simulink model "AsteroidImpact"  (R2020a)
settings: Solver=ode4  StartTime=0.0  StopTime=200  FixedStep=0.2  RelTol=1e-3
values from neighbouring files (symbols this model uses):
  K1 = 1.0e+03 *[-1.1353   -0.0611    0.0001   -0.0000;-0.0000   -0.0000    0.0000    1.0000]    [define_constants.m]    (also in setup_controller.m)
  K2 = 1.0e+03 *[-2.9174   -0.3964    0.0027    0.0000;0.0000    0.0000   -0.0000    0.0800]    [define_constants.m]    (also in setup_controller.m)
  MASS = 1000    [define_constants.m]
settings Model: Creator=KNMALE002  LastModifiedBy=Flaz
settings DataIOCC: SaveOutput=off  SignalLogging=off  DSMLogging=off  ReturnWorkspaceOutputs=off  TimeSaveName=simulation_time
settings DebuggingCC: ArithmeticOperatorsInVariantConditions=warning
settings SFSimCC: CustomCodeUndefinedFunction=UseInterfaceOnly

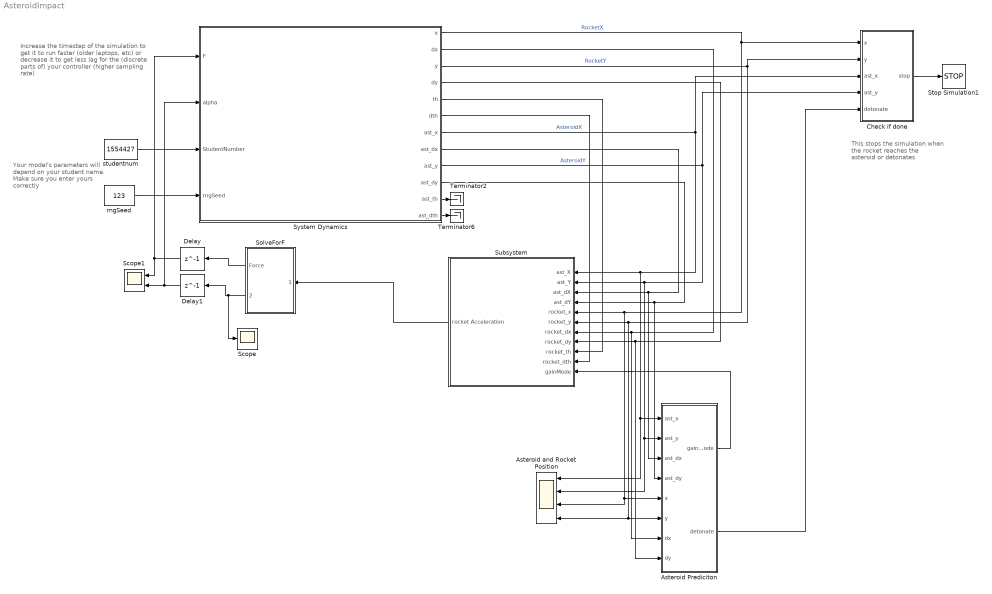
== system AsteroidImpact ==
  note: Increase the timestep of the simulation to get it to run faster (older laptops, etc) or decrease it to get less lag for the (discrete parts of) your controller (higher sampling rate)
  note: Your model's parameters will depend on your student name. Make sure you enter yours correctly
  note: This stops the simulation when the rocket reaches the asteroid or detonates
  Asteroid Prediciton : MATLAB Function  TreatAsAtomicUnit=on
  Asteroid and Rocket Position : Scope  NumInputPorts=4
  Check if done : MATLAB Function  TreatAsAtomicUnit=on
  Delay : Delay  DelayLength=1  InitialCondition=10000000000
  Delay1 : Delay  DelayLength=1
  Scope : Scope
  Scope1 : Scope  NumInputPorts=2
  SolveForF : MATLAB Function  TreatAsAtomicUnit=on
  Stop Simulation1 : Stop
  Subsystem : Subsystem
  System Dynamics : Subsystem  TreatAsAtomicUnit=on  mask{Value=2}
      mask prompts: Value "Enter mode (1, 2 or 3)"
      mask TypeOptions Value: ScenarioVar/Value
      mask Display: image('lander.jpg');
  Terminator2 : Terminator
  Terminator6 : Terminator
  rngSeed : Constant  Value=123
  studentnum : Constant  Value=1554427
  wires:
  studentnum/1 -> System Dynamics/3(StudentNumber)
  rngSeed/1 -> System Dynamics/4(rngSeed)
  System Dynamics/12(ast_dth) -> Terminator6/1
  System Dynamics/11(ast_th) -> Terminator2/1
  Check if done/1(stop) -> Stop Simulation1/1
  Delay1/1 -> Scope1/2, System Dynamics/2(alpha)
  Delay/1 -> Scope1/1, System Dynamics/1(F)
  System Dynamics/10(ast_dy) -> Asteroid Prediciton/4(ast_dy), Subsystem/4(ast_dY)
  SolveForF/1(Force) -> Delay/1
  SolveForF/2(angleAlpha) -> Scope/1, Delay1/1
  System Dynamics/1(x) -> Asteroid and Rocket Position/3, Asteroid Prediciton/5(x), Subsystem/5(rocket_x), Check if done/1(x)  "RocketX"
  System Dynamics/7(ast_x) -> Check if done/3(ast_x), Subsystem/1(ast_X), Asteroid Prediciton/1(ast_x), Asteroid and Rocket Position/1  "AsteroidX"
  System Dynamics/9(ast_y) -> Check if done/4(ast_y), Asteroid and Rocket Position/2, Asteroid Prediciton/2(ast_y), Subsystem/2(ast_Y)  "AsteroidY"
  System Dynamics/8(ast_dx) -> Asteroid Prediciton/3(ast_dx), Subsystem/3(ast_dX)
  System Dynamics/4(dy) -> Subsystem/8(rocket_dy), Asteroid Prediciton/8(dy)
  System Dynamics/2(dx) -> Asteroid Prediciton/7(dx), Subsystem/7(rocket_dx)
  System Dynamics/3(y) -> Check if done/2(y), Asteroid and Rocket Position/4, Asteroid Prediciton/6(y), Subsystem/6(rocket_y)  "RocketY"
  System Dynamics/5(th) -> Subsystem/9(rocket_th)
  System Dynamics/6(dth) -> Subsystem/10(rocket_dth)
  Subsystem/1(rocket Acceleration) -> SolveForF/1(rocketAcceleration)
  Asteroid Prediciton/1(gainMode) -> Subsystem/11(gainMode)
  Asteroid Prediciton/2(detonate) -> Check if done/5(detonate)

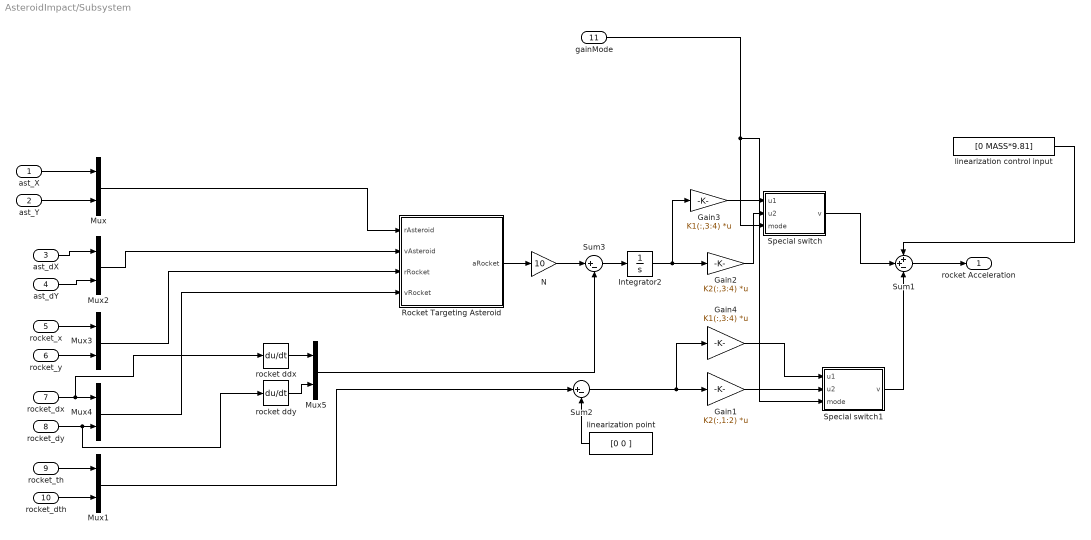
== system AsteroidImpact/Subsystem ==
  ast_X : Inport
  ast_Y : Inport  Port=2
  ast_dX : Inport  Port=3
  ast_dY : Inport  Port=4
  rocket_x : Inport  Port=5
  rocket_y : Inport  Port=6
  rocket_dx : Inport  Port=7
  rocket_dy : Inport  Port=8
  rocket_th : Inport  Port=9
  rocket_dth : Inport  Port=10
  gainMode : Inport  Port=11
  Gain1 : Gain  Gain=K2(:,1:2)  Multiplication=Matrix(K*u)
  Gain2 : Gain  Gain=K2(:,3:4)  Multiplication=Matrix(K*u)
  Gain3 : Gain  Gain=K1(:,3:4)  Multiplication=Matrix(K*u)
  Gain4 : Gain  Gain=K1(:,3:4)  Multiplication=Matrix(K*u)
  Integrator2 : Integrator
  Mux{,1..5} (6 alike) : Mux  Inputs=2
  N : Gain  Gain=10
  Rocket Targeting Asteroid : MATLAB Function  TreatAsAtomicUnit=on
  Special switch : MATLAB Function  TreatAsAtomicUnit=on
  Special switch1 : MATLAB Function  TreatAsAtomicUnit=on
  Sum1 : Sum  Inputs=++-
  Sum2 : Sum  Inputs=|+-
  Sum3 : Sum  Inputs=|+-
  linearization control input : Constant  Value=[0 MASS*9.81]
  linearization point : Constant  Value=[0 0 ]
  rocket ddx : Derivative
  rocket ddy : Derivative
  rocket Acceleration : Outport
  wires:
  Mux5/1 -> Sum3/2
  rocket_x/1 -> Mux3/1
  Sum3/1 -> Integrator2/1
  Mux2/1 -> Rocket Targeting Asteroid/2(vAsteroid)
  ast_X/1 -> Mux/1
  ast_Y/1 -> Mux/2
  ast_dX/1 -> Mux2/1
  ast_dY/1 -> Mux2/2
  rocket_dy/1 -> rocket ddy/1, Mux4/2
  rocket ddy/1 -> Mux5/2
  rocket_dx/1 -> rocket ddx/1, Mux4/1
  Rocket Targeting Asteroid/1(aRocket) -> N/1
  N/1 -> Sum3/1
  rocket ddx/1 -> Mux5/1
  rocket_y/1 -> Mux3/2
  Sum2/1 -> Gain4/1, Gain1/1
  Integrator2/1 -> Gain3/1, Gain2/1
  linearization point/1 -> Sum2/2
  Sum1/1 -> rocket Acceleration/1
  Mux3/1 -> Rocket Targeting Asteroid/3(rRocket)
  rocket_dth/1 -> Mux1/2
  rocket_th/1 -> Mux1/1
  linearization control input/1 -> Sum1/1
  Mux4/1 -> Rocket Targeting Asteroid/4(vRocket)
  Mux/1 -> Rocket Targeting Asteroid/1(rAsteroid)
  Mux1/1 -> Sum2/1
  Special switch/1(v) -> Sum1/2
  Gain2/1 -> Special switch/2(u2)
  Gain3/1 -> Special switch/1(u1)
  gainMode/1 -> Special switch1/3(mode), Special switch/3(mode)
  Special switch1/1(v) -> Sum1/3
  Gain1/1 -> Special switch1/2(u2)
  Gain4/1 -> Special switch1/1(u1)

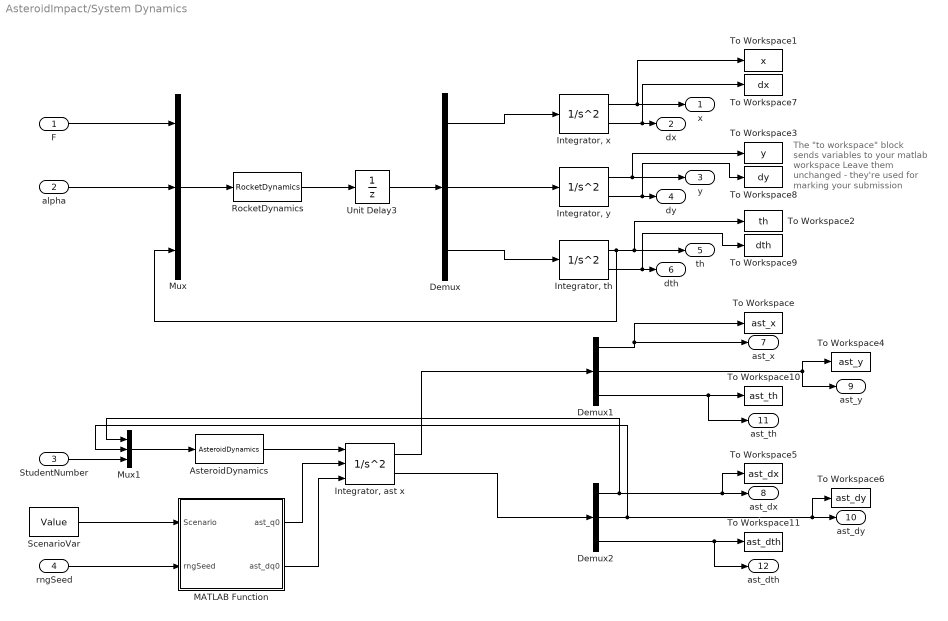
== system AsteroidImpact/System Dynamics ==
  note: The "to workspace" block sends variables to your matlab workspace
      |
      | Leave them unchanged - they're used for marking your submission
  F : Inport
  alpha : Inport  Port=2
  StudentNumber : Inport  Port=3
  rngSeed : Inport  Port=4
  AsteroidDynamics : MATLABFcn  MATLABFcn=AsteroidDynamics  OutputDimensions=3
  Demux : Demux  Outputs=3
  Demux1 : Demux  Outputs=3
  Demux2 : Demux  Outputs=3
  "Integrator, th" : SecondOrderIntegrator  ICX=0  ICDXDT=0
  "Integrator, x" : SecondOrderIntegrator  ICX=0
  "Integrator, y" : SecondOrderIntegrator  ICX=0
  "Integrator, ast x" : SecondOrderIntegrator  ICSourceX=external  ICX=x0  ICSourceDXDT=external
  MATLAB Function : MATLAB Function  TreatAsAtomicUnit=on
  Mux : Mux  Inputs=3
  Mux1 : Mux  Inputs=3
  RocketDynamics : MATLABFcn  MATLABFcn=RocketDynamics  Output1D=off
  ScenarioVar : Constant  Value=Value
  To Workspace : ToWorkspace  VariableName=ast_x  SampleTime=-1
  To Workspace1 : ToWorkspace  VariableName=x  SampleTime=-1
  To Workspace10 : ToWorkspace  VariableName=ast_th  SampleTime=-1
  To Workspace11 : ToWorkspace  VariableName=ast_dth  SampleTime=-1
  To Workspace2 : ToWorkspace  VariableName=th  SampleTime=-1
  To Workspace3 : ToWorkspace  VariableName=y  SampleTime=-1
  To Workspace4 : ToWorkspace  VariableName=ast_y  SampleTime=-1
  To Workspace5 : ToWorkspace  VariableName=ast_dx  SampleTime=-1
  To Workspace6 : ToWorkspace  VariableName=ast_dy  SampleTime=-1
  To Workspace7 : ToWorkspace  VariableName=dx  SampleTime=-1
  To Workspace8 : ToWorkspace  VariableName=dy  SampleTime=-1
  To Workspace9 : ToWorkspace  VariableName=dth  SampleTime=-1
  Unit Delay3 : UnitDelay  SampleTime=-1  HasFrameUpgradeWarning=on
  x : Outport  PortDimensions=1  VectorParamsAs1DForOutWhenUnconnected=off
  dx : Outport  Port=2  PortDimensions=1  VectorParamsAs1DForOutWhenUnconnected=off
  y : Outport  Port=3  PortDimensions=1  VectorParamsAs1DForOutWhenUnconnected=off
  dy : Outport  Port=4  PortDimensions=1  VectorParamsAs1DForOutWhenUnconnected=off
  th : Outport  Port=5  PortDimensions=1  VectorParamsAs1DForOutWhenUnconnected=off
  dth : Outport  Port=6  PortDimensions=1  VectorParamsAs1DForOutWhenUnconnected=off
  ast_x : Outport  Port=7  PortDimensions=1  VectorParamsAs1DForOutWhenUnconnected=off
  ast_dx : Outport  Port=8  PortDimensions=1  VectorParamsAs1DForOutWhenUnconnected=off
  ast_y : Outport  Port=9  PortDimensions=1  VectorParamsAs1DForOutWhenUnconnected=off
  ast_dy : Outport  Port=10  PortDimensions=1  VectorParamsAs1DForOutWhenUnconnected=off
  ast_th : Outport  Port=11  PortDimensions=1  VectorParamsAs1DForOutWhenUnconnected=off
  ast_dth : Outport  Port=12  PortDimensions=1  VectorParamsAs1DForOutWhenUnconnected=off
  wires:
  "Integrator, th"/1 -> th/1, To Workspace2/1, Mux/3
  Demux/1 -> "Integrator, x"/1
  Demux/2 -> "Integrator, y"/1
  Demux/3 -> "Integrator, th"/1
  "Integrator, x"/1 -> x/1, To Workspace1/1
  "Integrator, x"/2 -> To Workspace7/1, dx/1
  "Integrator, y"/2 -> To Workspace8/1, dy/1
  "Integrator, th"/2 -> To Workspace9/1, dth/1
  Mux/1 -> RocketDynamics/1
  RocketDynamics/1 -> Unit Delay3/1
  rngSeed/1 -> MATLAB Function/2(rngSeed)
  ScenarioVar/1 -> MATLAB Function/1(Scenario)
  F/1 -> Mux/1
  alpha/1 -> Mux/2
  Demux1/2 -> To Workspace4/1, ast_y/1
  Demux1/3 -> To Workspace10/1, ast_th/1
  Demux2/3 -> ast_dth/1, To Workspace11/1
  Mux1/1 -> AsteroidDynamics/1
  AsteroidDynamics/1 -> "Integrator, ast x"/1
  "Integrator, ast x"/1 -> Demux1/1
  "Integrator, ast x"/2 -> Demux2/1
  Demux1/1 -> To Workspace/1, ast_x/1
  Demux2/1 -> Mux1/1, To Workspace5/1, ast_dx/1
  Demux2/2 -> Mux1/2, To Workspace6/1, ast_dy/1
  MATLAB Function/1(ast_q0) -> "Integrator, ast x"/2
  MATLAB Function/2(ast_dq0) -> "Integrator, ast x"/3
  StudentNumber/1 -> Mux1/3
  Unit Delay3/1 -> Demux/1
  "Integrator, y"/1 -> y/1, To Workspace3/1

== matlab function AsteroidImpact/System Dynamics/MATLAB Function ==
  data: ast_q0 output; ast_dq0 output; Scenario input; rngSeed input
function [ast_q0, ast_dq0] = fcn(Scenario, rngSeed)
rng(rngSeed);

if (Scenario == 1)
    x0 = -3000;
    y0 =  5000;
    th0 =   0;
    dx0 = 182;
    dy0 = 0;
    dth0 = 0;

elseif (Scenario == 2)
    x0 = -2000 + rand_within_plus_minus(100);
    y0 = 4000 + rand_within_plus_minus(100); 
    th0 = 0;
    dx0 = 170;
    dy0 = 0;
    dth0 = 0.1;

elseif (Scenario == 3)
    x0 = -2500;
    y0 = 3000;
    th0 = 0;
    dx0 = 160;
    dy0 = 100;
    dth0 = deg2rad(rand_within_plus_minus(20)); % rad/sec

else
    error('You entered an invalid mode -- make sure Scenario = 1, 2 or 3')
end

ast_q0  = [ x0;  y0;  th0];
ast_dq0 = [dx0; dy0; dth0];

end

% calling rand_within_plus_minus(100) returns a number between -100 and 100
function n = rand_within_plus_minus(interval)
    n = (rand - 0.5) * 2 * interval;
end

== matlab function AsteroidImpact/Subsystem/Special switch ==
  data: u1 input; v output; u2 input; mode input
function v = fcn(u1,u2,mode)
if mode == 0
    v = u1;
else
    v=u2;
end

== matlab function AsteroidImpact/Subsystem/Rocket Targeting Asteroid ==
  data: rAsteroid input; aRocket output size=2; vAsteroid input; rRocket input; vRocket input
function aRocket = rocketNav(rAsteroid, vAsteroid, rRocket, vRocket)
% https://en.wikipedia.org/wiki/Proportional_navigation
% this produces an acceleration which the controller should track
R = rAsteroid - rRocket;
Rtemp = [R; 0];
Vr = vAsteroid - vRocket;
Vtemp = [Vr; 0];
omega = cross(Rtemp, Vtemp) / dot(Rtemp, Rtemp);
temp = cross(Vtemp, omega);
aRocket = temp(1:2);

== matlab function AsteroidImpact/Check if done ==
  data: x input; stop output; y input; ast_x input; ast_y input; detonate input
function stop = fcn(x, y, ast_x, ast_y, detonate)
    % given the signal to detonate
    if detonate == 1
        stop = 1;

    % rocket has hit the asteroid
    elseif norm([x; y] - [ast_x; ast_y]) < 100
        stop = 1;
    
    % rocket has hit the ground OR asteroid is close to they city
    elseif y < 0 || ast_y < 200
        stop = 1;
    
    else
        stop = 0;
    end
end

== matlab function AsteroidImpact/SolveForF ==
  data: rocketAcceleration input; Force output; angleAlpha output
function [Force, angleAlpha] = fcn(rocketAcceleration)
%ddx = -(Fx*cos(th) + Fy*sin(th))/mass
%ddy = -(g*mass - Fy*cos(th) + Fx*sin(th))/mass
%ddth = -(7*Fx)/(2*inertia)
%Fx = -F*sin(alpha+th)
%Fy = F*cos(alpha+th)
ddx = rocketAcceleration(1);
ddy = rocketAcceleration(2);


g = 9.81;
inertia = 36833.3333333333;
mass = 1000;


F = sqrt(ddx^2+ddy^2);
angleAlpha = atan(ddx/ddy);
Force = min(F,39000);

== matlab function AsteroidImpact/Asteroid Prediciton ==
  data: ast_x input; ast_y input; ast_dx input; ast_dy input; x input; gainMode output; y input; dx input; dy input; detonate output
function [gainMode, detonate] = prediction(ast_x,ast_y,ast_dx,ast_dy,x,y,dx,dy)
%check distance for detonate
cAst= 84.0811;
mAst = 10000;
g=9.81;
ddxAst = (cAst*sqrt(ast_dx^2+ast_dy^2))/mAst;
timeUntilAstatX0 = (-ast_dx+sqrt(2*ddxAst*(0-ast_x)+ast_dx^2))/ddxAst;

ddyAst = ((cAst*sqrt(ast_dx^2+ast_dy^2))/mAst)-g;
astYatX0 = ast_y+ast_dy*timeUntilAstatX0+0.5*ddyAst*timeUntilAstatX0^2;

if (astYatX0 > 3500) && (x <100)
    gainMode =0;
else
    gainMode =1;
end

distance = sqrt((ast_x-x)^2+(ast_y-y)^2);
if distance <= 150
    detonate =1;
else
    detonate =0;
end

== matlab function AsteroidImpact/Subsystem/Special switch1 ==
  data: u1 input; v output; u2 input; mode input
function v = fcn(u1,u2,mode)
if mode == 0
    v = u1;
else
    v=u2;
end
